simulink model "ROME_Main"  (R2025b)
settings: Solver=ode4  StartTime=0.0  StopTime=T_scaled  FixedStep=0.01  RelTol=1e-3  EnableMultiTasking=on
PostLoadFcn:
  | define_constants
StopFcn:
  | plotting
model workspace (MAT data in the model file):
  dddwad = 1
values from neighbouring files (symbols this model uses):
  alphas = [deg2rad(315), deg2rad(225), deg2rad(135), deg2rad(45)]    [define_constants.m]
  dist_scale = 1.0    (= 1)    [define_constants.m]
  elements = [1.4, 0.5, 0, 0, 0, 0]    [define_constants.m]
  EnableHardware = 0    [define_constants.m]
  EnableMotive = 0    [define_constants.m]
  Izz = (1/12)*m*(d^2+w^2)    (= 0.6075)    [define_constants.m]
  m = 18    [define_constants.m]
  mu = 1.0    (= 1)    [define_constants.m]
  r = 0.0762    [define_constants.m]
  time_scale = 0.40    (= 0.4)    [define_constants.m]
undefined symbols (not defined in the file or in its folder): omega, R
libraries: simulink x1
settings Model: Creator=ke350927  LastModifiedBy=benma
settings SolverCC: PositivePriorityOrder=on  AutoInsertRateTranBlk=on
settings DebuggingCC: UnderspecifiedInitializationDetection=Classic  MergeDetectMultiDrivingBlocksExec=none
settings HardwareCC: ProdBitPerLong=64.0  ProdHWDeviceType=Intel->x86-64 (Linux 64)
settings ModelReferenceCC: PropagateSignalLabelsOutOfModel=off
settings RTWCC: SystemTargetFile=sldrt.tlc  TemplateMakefile=sldrt.tmf  RTWCompilerOptimization=on  Description=Simulink Desktop Real-Time
settings CodeAppCC: MaxIdLength=95.0
settings STFCustomTargetCC: SystemTargetFile=sldrt.tlc  TargetLangStandard=C99 (ISO)  ModelReferenceCompliant=off  ConcurrentExecutionCompliant=off  MATLABClassNameForMDSCustomization=Simulink.SoftwareTarget.TargetSpecificTriggerConfigurationBase
settings SimscapeCC: SimscapeLogDataHistory=5000  SimscapeLogDecimation=1

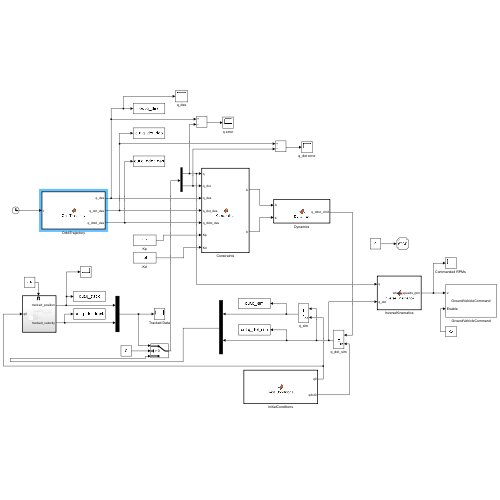
[thumbnail: Simulink's stored preview of the top-level diagram]
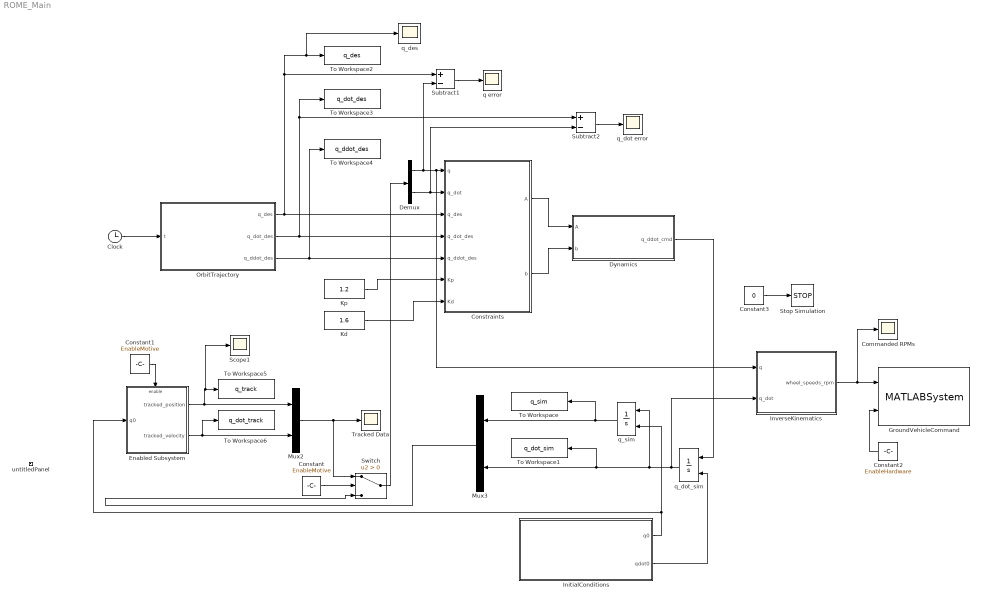
== system ROME_Main ==
  Clock : Clock
  "Commanded RPMs " : Scope
      settings: ActiveDisplayYMinimum=-87.74531  ActiveDisplayYMaximum=88.27276
  Constant : Constant  Value=EnableMotive
  Constant1 : Constant  Value=EnableMotive
  Constant2 : Constant  Value=EnableHardware
  Constant3 : Constant  Value=0
  Constraints : MATLAB Function  TreatAsAtomicUnit=on
  Demux : Demux  Outputs=2
  Dynamics : MATLAB Function  TreatAsAtomicUnit=on
  Enabled Subsystem : Subsystem  TreatAsAtomicUnit=on
  GroundVehicleCommand : MATLABSystem  Priority=2  System=GroundVehicleCommand  COMPort=COM3  BaudRate=115200  SimulateUsing=Interpreted execution
      mask Type: GroundVehicleCommand
  InitialConditions : MATLAB Function  TreatAsAtomicUnit=on
  InverseKinematics : MATLAB Function  TreatAsAtomicUnit=on
  Kd : Constant  Value=1.6
  Kp : Constant  Value=1.2
  Mux2 : Mux  Inputs=2
  Mux3 : Mux  Inputs=2
  OrbitTrajectory : MATLAB Function  TreatAsAtomicUnit=on
  Scope1 : Scope
      settings: ActiveDisplayYMinimum=-1.47357  ActiveDisplayYMaximum=1.85632
  Stop Simulation : Stop
  Subtract1 : Sum  Inputs=+-
  Subtract2 : Sum  Inputs=+-
  Switch : Switch  Criteria=u2 > Threshold  SaturateOnIntegerOverflow=off  InputSameDT=off
  To Workspace : ToWorkspace  VariableName=q_sim  SaveFormat=Timeseries  SampleTime=-1
  To Workspace1 : ToWorkspace  VariableName=q_dot_sim  SaveFormat=Timeseries  SampleTime=-1
  To Workspace2 : ToWorkspace  VariableName=q_des  SaveFormat=Timeseries  SampleTime=-1
  To Workspace3 : ToWorkspace  VariableName=q_dot_des  SaveFormat=Timeseries  SampleTime=-1
  To Workspace4 : ToWorkspace  VariableName=q_ddot_des  SaveFormat=Timeseries  SampleTime=-1
  To Workspace5 : ToWorkspace  VariableName=q_track  SaveFormat=Timeseries  SampleTime=-1
  To Workspace6 : ToWorkspace  VariableName=q_dot_track  SaveFormat=Timeseries  SampleTime=-1
  Tracked Data : Scope
      settings: ActiveDisplayYMinimum=-1.51772  ActiveDisplayYMaximum=1.20458
  q error : Scope
      settings: ActiveDisplayYMinimum=-0.2297  ActiveDisplayYMaximum=0.1407  DataLoggingVariableName=ScopeData2
  q_des : Scope
      settings: ActiveDisplayYMinimum=-2.51405  ActiveDisplayYMaximum=1.62649
  q_dot error : Scope
      settings: ActiveDisplayYMinimum=-0.75904  ActiveDisplayYMaximum=0.7358
  q_dot_sim : Integrator  InitialConditionSource=external  InitialCondition=[0, R*omega, 0]
  q_sim : Integrator  InitialConditionSource=external  InitialCondition=[R, 0, 0]
  untitledPanel : Subsystem  Tag=HiddenForWebPanel  IsWebBlockPanel=on
  wires:
  Clock/1 -> OrbitTrajectory/1(t)
  Constraints/1(A) -> Dynamics/1(A)
  Constraints/2(b) -> Dynamics/2(b)
  Switch/1 -> Demux/1
  q_sim/1 -> Mux3/1, To Workspace/1
  Dynamics/1(q_ddot_cmd) -> q_dot_sim/1
  Mux3/1 -> Switch/3
  InverseKinematics/1(wheel_speeds_rpm) -> "Commanded RPMs "/1, GroundVehicleCommand/1
  Enabled Subsystem/1(tracked_position) -> Scope1/1, To Workspace5/1, Mux2/1
  Enabled Subsystem/2(tracked_velocity) -> To Workspace6/1, Mux2/2
  Constant1/1 -> Enabled Subsystem/Enable
  Constant/1 -> Switch/2
  Constant2/1 -> GroundVehicleCommand/2
  Kp/1 -> Constraints/6(Kp)
  Kd/1 -> Constraints/7(Kd)
  Constant3/1 -> Stop Simulation/1
  Subtract1/1 -> q error/1
  OrbitTrajectory/1(q_des) -> Constraints/3(q_des), q_des/1, To Workspace2/1, Subtract1/1
  OrbitTrajectory/2(q_dot_des) -> Constraints/4(q_dot_des), To Workspace3/1, Subtract2/1
  OrbitTrajectory/3(q_ddot_des) -> Constraints/5(q_ddot_des), To Workspace4/1
  Demux/1 -> Subtract1/2, InverseKinematics/1(q), Constraints/1(q)
  Demux/2 -> Subtract2/2, Constraints/2(q_dot)
  InitialConditions/1(q0) -> q_sim/2, Enabled Subsystem/1(q0)
  InitialConditions/2(qdot0) -> q_dot_sim/2
  Mux2/1 -> Switch/1, Tracked Data/1
  q_dot_sim/1 -> InverseKinematics/2(q_dot), To Workspace1/1, Mux3/2, q_sim/1
  Subtract2/1 -> q_dot error/1

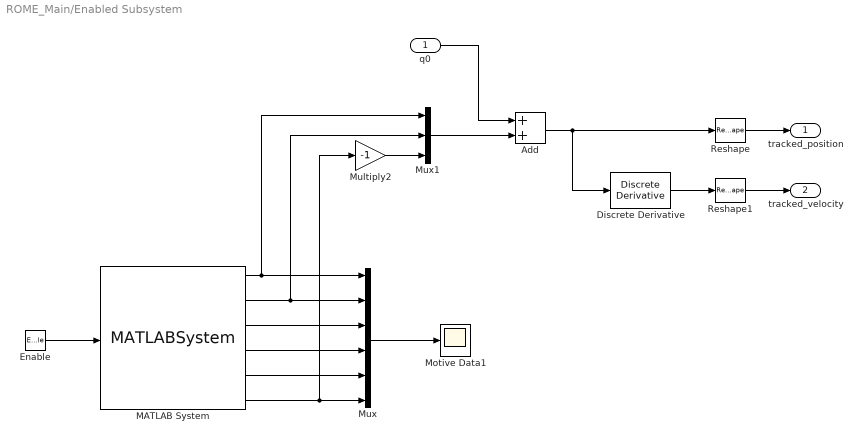
== system ROME_Main/Enabled Subsystem ==
  q0 : Inport
  Enable : EnablePort  ShowOutputPort=on
  Add : Sum
  Discrete Derivative : simulink/Discrete/Discrete Derivative  gainval=1.0  ICPrevScaledInput=0.0  OutMin=[]  OutMax=[]  OutDataType=fixdt(1, 16)  OutScaling=2^-10  DoSatur=off
  MATLAB System : MATLABSystem  Priority=1  System=MotiveData  RigidBodyID=1  HostIP=127.0.0.1  SimulateUsing=Interpreted execution
      mask Type: MotiveData
  Motive Data1 : Scope
      settings: ActiveDisplayYMinimum=-0.0048  ActiveDisplayYMaximum=0.32815  DataLoggingSaveFormat=Array
  Multiply2 : Gain  Gain=-1
  Mux : Mux  Inputs=6
  Mux1 : Mux  Inputs=3
  Reshape : Reshape  OutputDimensionality=Customize  OutputDimensions=[3, 1]
  Reshape1 : Reshape  OutputDimensionality=Customize  OutputDimensions=[3, 1]
  tracked_position : Outport
  tracked_velocity : Outport  Port=2
  wires:
  Discrete Derivative/1 -> Reshape1/1
  MATLAB System/4 -> Mux/4
  MATLAB System/3 -> Mux/3
  MATLAB System/5 -> Mux/5
  MATLAB System/6 -> Mux/6, Multiply2/1
  Mux/1 -> Motive Data1/1
  Enable/1 -> MATLAB System/1
  MATLAB System/2 -> Mux1/2, Mux/2
  MATLAB System/1 -> Mux1/1, Mux/1
  Multiply2/1 -> Mux1/3
  Reshape/1 -> tracked_position/1
  Reshape1/1 -> tracked_velocity/1
  Add/1 -> Discrete Derivative/1, Reshape/1
  Mux1/1 -> Add/2
  q0/1 -> Add/1

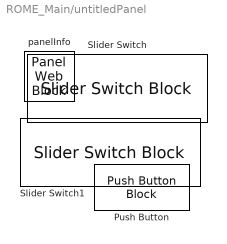
== system ROME_Main/untitledPanel ==
  Push Button : PushButtonBlock  Tag=HiddenForWebPanel  PanelInfo="{\"height\":87,\"left\":21,\"panelId\":\"panelId-a39fcf5c-14f9-48cf-a4ef-42f4a30cc727\",\"top\":169,\"type\":\"panelChild\",\"version\":\"2019b\",\"width\":175,\"zIndex\":1500006}"  ButtonText=STOP  Icon=Ex4  IconOnColor=[0.0, 0.39215686274509803, 0.0]  IconOffColor=[0.0, 1.0, 0.0]  OffValue=0.000000
  Slider Switch : SliderSwitchBlock  Tag=HiddenForWebPanel  PanelInfo="{\"height\":68,\"left\":18,\"panelId\":\"panelId-a39fcf5c-14f9-48cf-a4ef-42f4a30cc727\",\"top\":18,\"type\":\"panelChild\",\"version\":\"2019b\",\"width\":180,\"zIndex\":1500004}"
  Slider Switch1 : SliderSwitchBlock  Tag=HiddenForWebPanel  PanelInfo="{\"height\":68,\"left\":17,\"panelId\":\"panelId-a39fcf5c-14f9-48cf-a4ef-42f4a30cc727\",\"top\":93,\"type\":\"panelChild\",\"version\":\"2019b\",\"width\":180,\"zIndex\":1500008}"
  panelInfo : PanelWebBlock  Tag=HiddenForWebPanel  PanelInfo="{\"compacted\":false,\"height\":274,\"isActiveTab\":true,\"left\":1120,\"name\":\"Panel\",\"panelId\":\"panelId-a39fcf5c-14f9-48cf-a4ef-42f4a30cc727\",\"popoutData\":{\"height\":0,\"left\":0,\"maximized\":false,\"top\":0,\"width\":0},\"popoutMode\":\"component\",\"tabIndex\":0,\"tabbedSetId\":\"tabbedSet7305451321\",\"top\":89,\"type\":\"panel\",\"version\":\"2019b\",\"visible\":true,\"width\":214,\"zIndex\":1500002}"  PanelSnapshot=<binary blob, 7196 chars, not shown>

== matlab function ROME_Main/Dynamics ==
  data: A input; b input; q_ddot_cmd output size=[3 1]; m parameter; Izz parameter
function q_ddot_cmd = Dynamics(A,b, m, Izz)

M = [m 0 0; 
     0 m 0; 
     0 0 Izz];

Q = [0; 0; 0];

a = M\Q;

M_complex = complex(M);
Q_c_complex = (M_complex^(1/2)) * (pinv(A * (M_complex^(-1/2)))) * (b - A * a);
Q_c = real(Q_c_complex);
 
q_ddot_cmd = M\Q + M\Q_c;

end

== matlab function ROME_Main/Constraints ==
  data: q input; q_dot input; q_des input; q_dot_des input; q_ddot_des input; Kp input; Kd input; A output; b output
function [A, b] = Constraints(q, q_dot, q_des, q_dot_des, q_ddot_des, Kp, Kd)

    A = [1 0 0;
         0 1 0;
         0 0 1];

    b = q_ddot_des + Kd.*(q_dot_des - q_dot) + Kp.*(q_des - q);
end

== matlab function ROME_Main/InverseKinematics ==
  data: q input; q_dot input; wheel_speeds_rpm output; alphas parameter; r parameter
function wheel_speeds_rpm = InverseKinematics(q, q_dot, alphas, r)
% wheel_speeds_rpm = [0;0;0;0];

theta = q(3);

R_transpose = [ cos(theta), sin(theta), 0;
                   -sin(theta), cos(theta), 0;
                    0,          0,          1];

q_dot_body = R_transpose * q_dot;

%% Source: https://eprints.undip.ac.id/79371/1/C14-Development_of_Omni-Wheeled_Mobile_Robot_Based-on_Inverse_Kinematics_and_Odometry.pdf

%% IK transform matrix from body velocities to angular wheel speeds
A = (1/r) * [sin(alphas); 
             cos(alphas); 
             repmat(r, 1, 4)]; 

wheel_speeds_rad = A.'*q_dot_body; % Transpose
wheel_speeds_rpm = wheel_speeds_rad * 60/(2*pi);

end

== matlab function ROME_Main/OrbitTrajectory ==
  data: q_des output; t input; q_dot_des output; q_ddot_des output; elements parameter; mu parameter; time_scale parameter; dist_scale parameter
function [q_des, q_dot_des, q_ddot_des] = OrbitTrajectory(t, elements, mu, time_scale, dist_scale)
    % elements = [a, e, i, Omega, omega, nu0]
    
    % Extract and Scale Elements
    a_raw = elements(1);
    e = elements(2);
    i = elements(3);
    Omega = elements(4);
    omega = elements(5);
    nu0 = elements(6); 
    
    a = a_raw * dist_scale;
    scaled_t = t * time_scale;
    
    % Solve for current True Anomaly (nu)
    p = a * (1 - e^2);
    n = sqrt(mu / a^3);
    
    M = n * scaled_t; 
    
    % Iterative Newton-Raphson for Eccentric Anomaly
    E = M; 
    for j = 1:5
        E = E - (E - e*sin(E) - M) / (1 - e*cos(E));
    end
    
    % Solve for current True Anomaly (nu)
    p = a * (1 - e^2);
    n = sqrt(mu / a^3);
    
    % Convert nu0 to an initial Eccentric Anomaly (E0)
    E0 = 2 * atan(sqrt((1-e)/(1+e)) * tan(nu0/2));
    % Convert E0 to an initial Mean Anomaly (M0)
    M0 = E0 - e*sin(E0);
    
    % Current Mean Anomaly is initial + progress
    M = M0 + (n * scaled_t); 
    
    % Iterative Newton-Raphson for Eccentric Anomaly (E)
    E = M; 
    for j = 1:5
        E = E - (E - e*sin(E) - M) / (1 - e*cos(E));
    end
    
    % True Anomaly calculation (Don't add nu0 here!)
    nu = 2 * atan2(sqrt(1+e)*sin(E/2), sqrt(1-e)*cos(E/2));
    
    % Perifocal Position and Velocity (PQW Frame)
    r_mag = p / (1 + e*cos(nu));
    
    r_pqw = [r_mag * cos(nu); 
             r_mag * sin(nu); 
             0];
         
    v_pqw = sqrt(mu/p) * [-sin(nu); 
                          e + cos(nu); 
                          0] * time_scale; 

    % Perifocal Acceleration
    accel_pqw = (-mu / r_mag^3) * r_pqw * (time_scale^2);

    % Rotation Matrix (Perifocal to ECI)
    cO = cos(Omega); sO = sin(Omega);
    co = cos(omega); so = sin(omega);
    ci = cos(i);     si = sin(i);
    
    R = [cO*co-sO*so*ci, -cO*so-sO*co*ci,  sO*si;
         sO*co+cO*so*ci, -sO*so+cO*co*ci, -cO*si;
         so*si,           co*si,           ci];

    % Transform to ECI
    r_eci = R * r_pqw;
    v_eci = R * v_pqw;
    a_eci = R * accel_pqw;

    % Project to 2D Floor (x, y, theta)
    x = r_eci(1);
    y = r_eci(2);
    
    % Get the raw angle (-pi to pi)
    theta_raw = atan2(v_eci(2), v_eci(1));
    
    % Calculate the "Mean Motion" progress
    total_progress = n * scaled_t; 
    
    % Offset the raw angle based on progress
    revolutions = floor((total_progress + nu0) / (2*pi));
    theta = theta_raw + (revolutions * 2*pi);
    
    % Small logic gate to handle the jump-point precisely
    if (theta - total_progress) < -pi
        theta = theta + 2*pi;
    elseif (theta - total_progress) > pi
        theta = theta - 2*pi;
    end
    % Mismatch between Math (0=East) and Robot (0=North)
    heading_offset = -pi/2;
    theta = theta + heading_offset;
    
    % Heading tangent to the velocity vector
    x_dot = v_eci(1);
    y_dot = v_eci(2);
    
    % Angular velocity calculation (The "Derivative")
    v_sq = x_dot^2 + y_dot^2;
    if v_sq > 1e-6
        % This formula gives the continuous derivative of atan2(y,x)
        % theta_dot = (x*y_ddot - y*x_ddot) / (x^2 + y^2)
        theta_dot = (v_eci(1)*a_eci(2) - v_eci(2)*a_eci(1)) / v_sq;
    else
        theta_dot = 0;
    end

    % Assign outputs
    % q_des = [x; y; -theta]; 
    % q_dot_des = [x_dot; y_dot; -theta_dot];
    % q_ddot_des = [a_eci(1); a_eci(2); 0]; 
    q_des = [x; y; 0]; 
    q_dot_des = [x_dot; y_dot; 0];
    q_ddot_des = [a_eci(1); a_eci(2); 0]; 
end

== matlab function ROME_Main/InitialConditions ==
  data: q0 output; qdot0 output; elements parameter; mu parameter; time_scale parameter; dist_scale parameter
function [q0, qdot0] = InitialConditions(elements, mu, time_scale, dist_scale)
    % elements = [a, e, i, Omega, omega, nu0]
    
    % 1. Extract and Scale
    a = elements(1) * dist_scale;
    e = elements(2);
    i = elements(3);
    Omega = elements(4);
    omega = elements(5);
    nu0 = elements(6); % Starting position in the orbit
    
    % 2. Constant Parameters
    p = a * (1 - e^2);
    
    % 3. Initial Position in Perifocal Frame (PQW)
    r_mag = p / (1 + e * cos(nu0));
    r_pqw = [r_mag * cos(nu0); 
             r_mag * sin(nu0); 
             0];
         
    % 4. Initial Velocity in Perifocal Frame (PQW)
    % Note: Velocity must be scaled by time_scale to match your propagator
    v_pqw = sqrt(mu / p) * [-sin(nu0); 
                           (e + cos(nu0)); 
                            0] * time_scale;

    % 5. Acceleration in PQW (Needed for initial theta_dot)
    accel_pqw = (-mu / r_mag^3) * r_pqw * (time_scale^2);

    % 6. Rotation Matrix (Perifocal to ECI)
    cO = cos(Omega); sO = sin(Omega);
    co = cos(omega); so = sin(omega);
    ci = cos(i);     si = sin(i);

    T = [cO*co-sO*so*ci, -cO*so-sO*co*ci,  sO*si;
         sO*co+cO*so*ci, -sO*so+cO*co*ci, -cO*si;
         so*si,           co*si,           ci];

    % 7. Transform to ECI Frame
    r_eci = T * r_pqw;
    v_eci = T * v_pqw;
    a_eci = T * accel_pqw;

    % 8. Project to 2D State (x, y, theta)
    x0 = r_eci(1);
    y0 = r_eci(2);
    theta0 = atan2(v_eci(2), v_eci(1));

    % Mismatch between Math (0=East) and Robot (0=North)
    heading_offset = -pi/2;
    theta0 = theta0 + heading_offset;

    x_dot0 = v_eci(1);
    y_dot0 = v_eci(2);
    
    % Angular velocity of the heading vector (theta_dot)
    % Derived from the 2D cross product of velocity and acceleration
    v_mag_sq = v_eci(1)^2 + v_eci(2)^2;
    if v_mag_sq > 1e-6
        theta_dot0 = (v_eci(1)*a_eci(2) - v_eci(2)*a_eci(1)) / v_mag_sq;
    else
        theta_dot0 = 0;
    end

    % 9. Form Output Vectors
    % q0 = [x0; y0; -theta0];
    % qdot0 = [x_dot0; y_dot0; -theta_dot0];
    q0 = [x0; y0; 0];
    qdot0 = [x_dot0; y_dot0; 0];
end
